simulink model "Pendulum_nlmodel_link1"  (R2016a)
settings: Solver=ode45  StartTime=0.0  StopTime=10  RelTol=1e-3
model workspace: external: MATLAB File D:\Documenten\Biomedical Engineering\2016-2017\Control Systems Lab\Lab sessie 1\CSL\Dick\params.m (data not in the file)
values from neighbouring files (symbols this model uses):
  x0 = [0.5*pi+0.001 -0.001 0 0 0]    [nonlinid_pendulum.m]
undefined symbols (not defined in the file or in its folder): input_costfun, k_m_hat, tau_e_hat
settings Model: Creator=Nathan  LastModifiedBy=Dick
settings DataIOCC: InitialState=states  LimitDataPoints=on  SaveFormat=Array
settings DebuggingCC: AllowSymbolicDim=off
settings HardwareCC: ProdBitPerPointer=32  ProdLargestAtomicFloat=None  ProdIntDivRoundTo=Undefined  ProdEndianess=Unspecified  ProdWordSize=32  ProdHWDeviceType=32-bit Generic
settings ModelReferenceCC: PropagateSignalLabelsOutOfModel=off
settings ConfigComp: CovModelRefEnable=Off

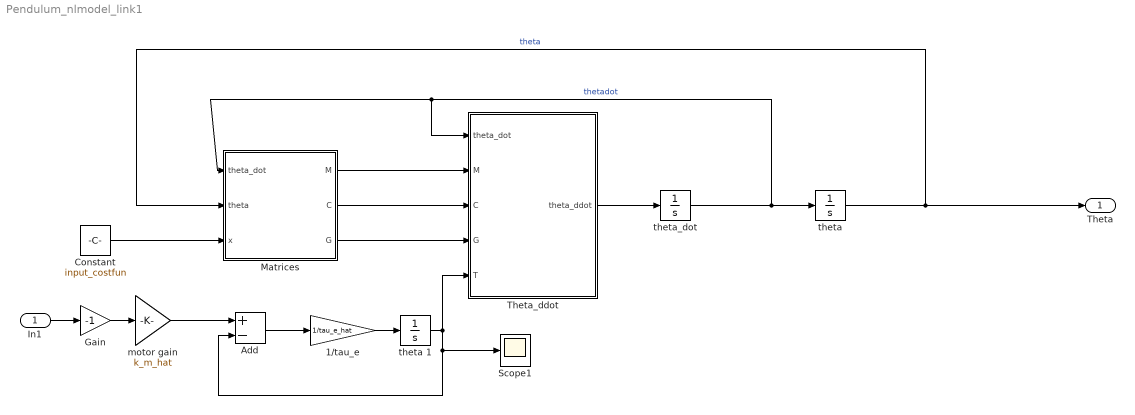
== system Pendulum_nlmodel_link1 ==
  In1 : Inport
  "1/tau_e " : Gain  Gain=1/tau_e_hat
  Add : Sum  Inputs=+-
  Constant : Constant  Value=input_costfun  SampleTime=-1
  Gain : Gain  Gain=-1
  Matrices : MATLAB Function  TreatAsAtomicUnit=on
  Scope1 : Scope
  "Theta_ddot " : MATLAB Function  TreatAsAtomicUnit=on
  "motor gain " : Gain  Gain=k_m_hat
  "theta " : Integrator  InitialCondition=[x0(1) x0(2)]
  theta 1 : Integrator  InitialCondition=x0(5)  ContinuousStateAttributes='torque'
  "theta_dot " : Integrator  InitialCondition=[x0(3) x0(4)]
  Theta : Outport
  wires:
  "theta "/1 -> Theta/1, Matrices/2(theta)  "theta"
  "theta_dot "/1 -> "theta "/1, "Theta_ddot "/1(theta_dot), Matrices/1(theta_dot)  "thetadot"
  "Theta_ddot "/1(theta_ddot) -> "theta_dot "/1
  Matrices/3(G) -> "Theta_ddot "/4(G)
  Matrices/2(C) -> "Theta_ddot "/3(C)
  Matrices/1(M) -> "Theta_ddot "/2(M)
  theta 1/1 -> Scope1/1, Add/2, "Theta_ddot "/5(T)
  "1/tau_e "/1 -> theta 1/1
  Add/1 -> "1/tau_e "/1
  "motor gain "/1 -> Add/1
  Constant/1 -> Matrices/3(x)
  Gain/1 -> "motor gain "/1
  In1/1 -> Gain/1

== matlab function Pendulum_nlmodel_link1/Theta_ddot  ==
  data: theta_dot input; M input; C input; G input; theta_ddot output; T input
function theta_ddot = fcn(theta_dot,M,C,G,T)
theta_ddot = [0;0];

theta_ddot = M\[T;0] - M\C*theta_dot - M\G;

== matlab function Pendulum_nlmodel_link1/Matrices ==
  data: theta_dot input; theta input; M output; C output; G output; x input
function [M, C, G] = fcn(theta_dot, theta, x)

M = zeros(2);
C = zeros(2);
G = [0;0];

l1 = 0.1;
m1 = 0.125;
c1 = -0.04;
I1 = 0.074;

b1 = x(1);
b2 = x(2);

g = 9.81; 
% l1 = 0.1;
l2 = 0.1;
% m1 = 0.125;
m2 = 0.05;
% c1 = -0.04; % Keeping it negative results in no motion at all, -0.04 or + 0.04?
c2 = 0.06;
% I1 = 0.074;
I2 = 0.00012;
% b1 = 4.8;
% b2 = 0.0002;

P1 = m1*c1^2+m2*l1^2+I1;
P2 = m2*c2^2+ I2;
P3 = m2*l1*c2;
g1 = (m1*c1+m2*l1)*g;
g2 = m2*c2*g;

M = [(P1 + P2 + 2*P3*cos(theta(2)))               (P2 + P3*cos(theta(2))) ;
     (P2 + P3*cos(theta(2)))                       P2                   ];
 
 
C = [(b1 - P3*theta_dot(2)*sin(theta(2)))           (-P3*(theta_dot(1)+theta_dot(2))*sin(theta(2))) ;
     (P3*theta_dot(1)*sin(theta(2)))                 b2                                      ];
     
G = [(-g1*sin(theta(1))-g2*sin(theta(1) + theta(2))) ;
      -g2*sin(theta(1)+theta(2))                   ];
